simulink model "TrafegabilidadeVerticalAtivo"  (R2018a)
settings: Solver=ode3  StartTime=0.0  StopTime=60  FixedStep=0.0001  RelTol=1e-3
values from neighbouring files (symbols this model uses):
  a1 = 1    [Algoritmo_gen.m]    (also in Parametros_dissertacao_Jeff.m = 1.99; custo_gen.m)
  a2 = 100    [Algoritmo_gen.m]    (also in Parametros_dissertacao_Jeff.m = 1.988; custo_gen.m)
  b1 = 0.675    [Parametros_dissertacao_Jeff.m]
  b2 = 0.675    [Parametros_dissertacao_Jeff.m]
  bp11 = 2660    [Parametros_Susp_Ativa_GALQR.m]    (also in Parametros_dissertacao_Jeff.m)
  bp2 = 2660    [Parametros_dissertacao_Jeff.m]
  bp3 = 2660    [Parametros_dissertacao_Jeff.m]
  bs11 = 24500    [Parametros_Susp_Ativa_GALQR.m]    (also in Parametros_dissertacao_Jeff.m)
  bs2 = 10000    [Parametros_dissertacao_Jeff.m]
  bs3 = 8000    [Parametros_dissertacao_Jeff.m]
  d = 50    [Parametros_dissertacao_Jeff.m]
  fr = 0.01    [Parametros_dissertacao_Jeff.m]
  g = 9.81    [Parametros_dissertacao_Jeff.m]
  h = eig(A_cl2)    [Algoritmo_gen.m]    (also in Parametros_dissertacao_Jeff.m = 0.3; custo_gen.m)
  hcg = 1.359    [Parametros_dissertacao_Jeff.m]
  Ibyy = 66.080    (= 66.08)    [Parametros_dissertacao_Jeff.m]
  Iyy = 284800    [Parametros_dissertacao_Jeff.m]
  kp11 = 870000    [Parametros_Susp_Ativa_GALQR.m]    (also in Parametros_dissertacao_Jeff.m)
  kp2 = 770700    [Parametros_dissertacao_Jeff.m]
  kp3 = 770700    [Parametros_dissertacao_Jeff.m]
  ks11 = 55000    [Parametros_Susp_Ativa_GALQR.m]    (also in Parametros_dissertacao_Jeff.m)
  ks2 = 3220000    [Parametros_dissertacao_Jeff.m]
  ks3 = 2740000    [Parametros_dissertacao_Jeff.m]
  L = 7    [Parametros_dissertacao_Jeff.m]
  m11 = 490    [Parametros_Susp_Ativa_GALQR.m]    (also in Parametros_dissertacao_Jeff.m)
  m2 = 4500    [Algoritmo_gen.m]    (also in Parametros_dissertacao_Jeff.m = 1700; custo_gen.m; n1sistema.m = s(2))
  m3 = 1700    [Parametros_dissertacao_Jeff.m]
  ms = 18470    [Parametros_dissertacao_Jeff.m]
  ms_b = 200    [Parametros_dissertacao_Jeff.m]
  mv = 22560    [Parametros_dissertacao_Jeff.m]
  r_est = 0.542    [Parametros_dissertacao_Jeff.m]
  r_ind = (20*25.4/2+0.5*0.85*395)/1000    (= 0.421875)    [Parametros_dissertacao_Jeff.m]
(part 1 of 2)
settings Model: Creator=MA  LastModifiedBy=jeffersongomes
settings CodeAppCC: StateflowObjectComments=on
settings SimscapeCC: SimscapeNormalizeSystem=off

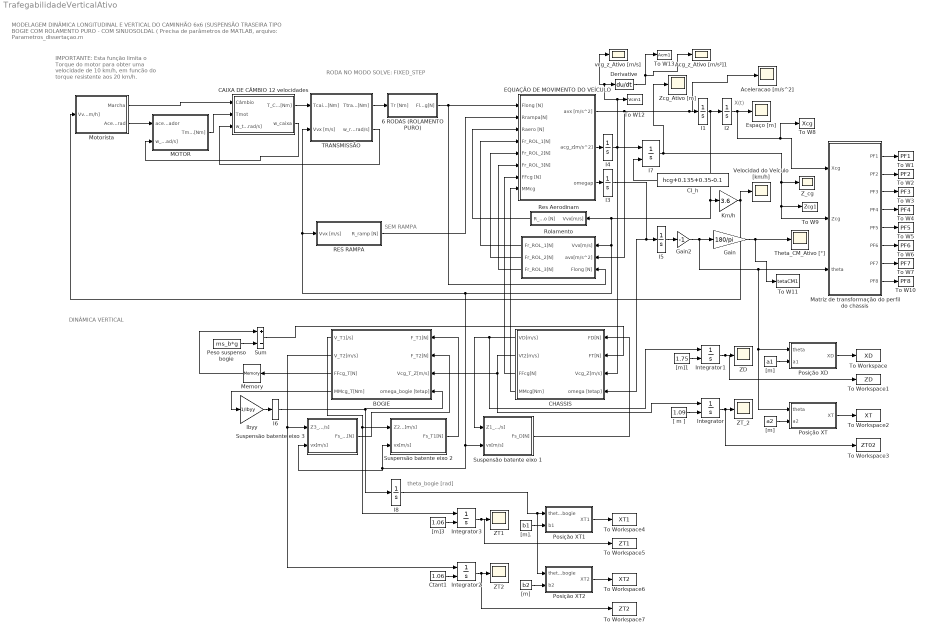
== system TrafegabilidadeVerticalAtivo ==
  note: theta_bogie [rad]
  note: SEM RAMPA
  note: RODA NO MODO SOLVE: FIXED_STEP
  note: DINÂMICA VERTICAL
  note: MODELAGEM DINÂMICA LONGITUDINAL E VERTICAL DO CAMINHÃO 6x6 (SUSPENSÃO TRASEIRA TIPO BOGIE COM ROLAMENTO PURO - COM SINUOSOLDAL
      | ( Precisa de parâmetros de MATLAB, arquivo: Parametros_dissertaçao.m
  note: X(t)
  note: IMPORTANTE:
      | Esta função limita o Torque do motor para obter uma velocidade
      | de 10 km/h, em funcão do torque resistente
      | aos 20 km/h.
  6 RODAS (ROLAMENTO PURO) : Subsystem
  Aceleracao [m/s^2] : Scope
  Acg_z_Ativo [m/s²]1 : Scope
  BOGIE : Subsystem
  CAIXA DE CÂMBIO 12 velocidades : Subsystem
  CHASSIS : Subsystem
  CI_h : Constant  Value=hcg+0.135+0.35-0.1
  Ctant1 : Constant  Value=1.06
  Derivative : Derivative
  EQUAÇÃO DE MOVIMENTO DO VEÍCULO : Subsystem
  Espaço [m] : Scope
  Gain : Gain  Gain=180/pi
  Gain2 : Gain  Gain=-1
  I1 : Integrator
  I{2..4,6} (4 alike) : Integrator  InitialCondition=eps
  I5 : Integrator  InitialCondition=-8*pi/180
  I7 : Integrator  InitialConditionSource=external  InitialCondition=1.25
  I8 : Integrator
  Ibyy : Gain  Gain=1/Ibyy
  Integrator{,1..3} (4 alike) : Integrator  InitialConditionSource=external
  Km/h : Gain  Gain=3.6
  MOTOR : Subsystem
  Matriz de transformação do perfil do chassis : MATLAB Function  TreatAsAtomicUnit=on
  Memory : Memory
  Motorista : Subsystem
  Peso suspenso bogie : Constant  Value=ms_b*g
  Posição XD : MATLAB Function  TreatAsAtomicUnit=on
  Posição XT : MATLAB Function  TreatAsAtomicUnit=on
  Posição XT1 : MATLAB Function  TreatAsAtomicUnit=on
  Posição XT2 : MATLAB Function  TreatAsAtomicUnit=on
  RES RAMPA : Subsystem
  Res Aerodinam : Subsystem
  Rolamento : Subsystem
  Sum : Sum  Inputs=+|-
  Suspensão batente eixo 1 : Subsystem
  Suspensão batente eixo 2 : Subsystem
  Suspensão batente eixo 3 : Subsystem
  TRANSMISSÃO : Subsystem
  Theta_CM_Ativo [°] : Scope
  To W1 : ToWorkspace  VariableName=PF1  SampleTime=-1
      settings: Save2DSignal=2-D array (concatenate along first dimension)
  To W10 : ToWorkspace  VariableName=PF8  SampleTime=-1
      settings: Save2DSignal=2-D array (concatenate along first dimension)
  To W11 : ToWorkspace  VariableName=tetaCM1  SampleTime=-1
      settings: Save2DSignal=2-D array (concatenate along first dimension)
  To W12 : ToWorkspace  VariableName=Vcm1  SampleTime=-1
      settings: Save2DSignal=2-D array (concatenate along first dimension)
  To W13 : ToWorkspace  VariableName=Acm1  SampleTime=-1
      settings: Save2DSignal=2-D array (concatenate along first dimension)
  To W2 : ToWorkspace  VariableName=PF2  SampleTime=-1
      settings: Save2DSignal=2-D array (concatenate along first dimension)
  To W3 : ToWorkspace  VariableName=PF3  SampleTime=-1
      settings: Save2DSignal=2-D array (concatenate along first dimension)
  To W4 : ToWorkspace  VariableName=PF4  SampleTime=-1
      settings: Save2DSignal=2-D array (concatenate along first dimension)
  To W5 : ToWorkspace  VariableName=PF5  SampleTime=-1
      settings: Save2DSignal=2-D array (concatenate along first dimension)
  To W6 : ToWorkspace  VariableName=PF6  SampleTime=-1
      settings: Save2DSignal=2-D array (concatenate along first dimension)
  To W7 : ToWorkspace  VariableName=PF7  SampleTime=-1
      settings: Save2DSignal=2-D array (concatenate along first dimension)
  To W8 : ToWorkspace  VariableName=Xcg  SampleTime=-1
      settings: Save2DSignal=2-D array (concatenate along first dimension)
  To W9 : ToWorkspace  VariableName=Zcg1  SampleTime=-1
      settings: Save2DSignal=2-D array (concatenate along first dimension)
  To Workspace : ToWorkspace  VariableName=XD  SampleTime=-1
      settings: Save2DSignal=2-D array (concatenate along first dimension)
  To Workspace1 : ToWorkspace  VariableName=ZD  SampleTime=-1
      settings: Save2DSignal=2-D array (concatenate along first dimension)
  To Workspace2 : ToWorkspace  VariableName=XT  SampleTime=-1
      settings: Save2DSignal=2-D array (concatenate along first dimension)
  To Workspace3 : ToWorkspace  VariableName=ZT02  SampleTime=-1
      settings: Save2DSignal=2-D array (concatenate along first dimension)
  To Workspace4 : ToWorkspace  VariableName=XT1  SampleTime=-1
      settings: Save2DSignal=2-D array (concatenate along first dimension)
  To Workspace5 : ToWorkspace  VariableName=ZT1  SampleTime=-1
      settings: Save2DSignal=2-D array (concatenate along first dimension)
  To Workspace6 : ToWorkspace  VariableName=XT2  SampleTime=-1
      settings: Save2DSignal=2-D array (concatenate along first dimension)
  To Workspace7 : ToWorkspace  VariableName=ZT2  SampleTime=-1
      settings: Save2DSignal=2-D array (concatenate along first dimension)
  Velocidad do Veículo [km/h] : Scope
  ZD : Scope
  ZT1 : Scope
  ZT2 : Scope
  ZT_2 : Scope
  Z_cg : Scope
  Zcg_Ativo [m] : Scope
  "[ m ] " : Constant  Value=1.09
  "[m]" : Constant  Value=a1
  "[m] " : Constant  Value=a2
  "[m]  " : Constant  Value=b2
  "[m]." : Constant  Value=b1
  "[m]1" : Constant  Value=1.75
  "[m]3" : Constant  Value=1.06
  vcg_z_Ativo [m/s] : Scope
  wires:
  I2/1 -> Matriz de transformação do perfil do chassis/1(Xcg), To W8/1, Espaço [m]/1
  MOTOR/1(Tmot[Nm]) -> CAIXA DE CÂMBIO 12 velocidades/2(Tmot)
  Motorista/1(Marcha) -> CAIXA DE CÂMBIO 12 velocidades/1(Câmbio)
  CAIXA DE CÂMBIO 12 velocidades/2(w_caixa) -> MOTOR/2(w_Trans [rad/s])
  CAIXA DE CÂMBIO 12 velocidades/1(T_Caixa[Nm]) -> TRANSMISSÃO/1(Tcaixa[Nm])
  TRANSMISSÃO/2(w_roda[rad/s]) -> CAIXA DE CÂMBIO 12 velocidades/3(w_trans[rad/s])
  RES RAMPA/1(R_ramp [N]) -> EQUAÇÃO DE MOVIMENTO DO VEÍCULO/2(Rrampa[N])
  Rolamento/1(Fr_ROL_1[N]) -> EQUAÇÃO DE MOVIMENTO DO VEÍCULO/4(Fr_ROL_1[N])
  TRANSMISSÃO/1(Ttrans[Nm]) -> 6 RODAS (ROLAMENTO PURO)/1(Tr [Nm])
  6 RODAS (ROLAMENTO PURO)/1(Flong[N]) -> EQUAÇÃO DE MOVIMENTO DO VEÍCULO/1(Flong [N]), Rolamento/3(Flong [N])
  EQUAÇÃO DE MOVIMENTO DO VEÍCULO/1(avx [m/s^2]) -> Aceleracao [m/s^2]/1, I1/1, Rolamento/2(avx[m/s^2])
  EQUAÇÃO DE MOVIMENTO DO VEÍCULO/3(omegap) -> I3/1
  I3/1 -> I5/1, CHASSIS/4(omega [tetap])
  EQUAÇÃO DE MOVIMENTO DO VEÍCULO/2(acg_z[m/s^2]) -> I4/1
  I4/1 -> I7/1, CHASSIS/3("Vcg_Z[m/s] "), vcg_z_Ativo [m/s]/1, Derivative/1, To W12/1
  CHASSIS/3("FFcg[N] ") -> EQUAÇÃO DE MOVIMENTO DO VEÍCULO/7(FFcg [N])
  CHASSIS/4(MMcg[Nm]) -> EQUAÇÃO DE MOVIMENTO DO VEÍCULO/8(MMcg)
  Suspensão batente eixo 1/1(Fs_D[N]) -> CHASSIS/1(FD[N])
  Gain/1 -> To W11/1, Theta_CM_Ativo [°]/1
  Suspensão batente eixo 2/1(Fs_T1[N]) -> BOGIE/1(F_T1[N])
  Suspensão batente eixo 3/1(Fs_T2[N]) -> BOGIE/2(F_T2[N])
  BOGIE/1("V_T1[/s] ") -> Integrator3/1, Suspensão batente eixo 2/1(Z2_p[m/s])
  BOGIE/2("V_T2[m/s] ") -> Integrator2/1, Suspensão batente eixo 3/1(Z3_p[m/s])
  Peso suspenso bogie/1 -> Sum/2
  BOGIE/3("FFcg_T[N] ") -> Memory/1
  Sum/1 -> CHASSIS/2(FT[N])
  BOGIE/4(MMcg_T[Nm]) -> Ibyy/1
  Ibyy/1 -> I6/1
  I1/1 -> I2/1, Res Aerodinam/1(Vvx[m/s]), RES RAMPA/1(Vvx [m/s]), TRANSMISSÃO/2(Vvx [m/s]), Suspensão batente eixo 3/2(vx[m/s]), Suspensão batente eixo 2/2(vx[m/s]), Suspensão batente eixo 1/2(vx[m/s]), Rolamento/1(Vvx[m/s]), Km/h/1
  Integrator/1 -> To Workspace3/1, ZT_2/1
  "[ m ] "/1 -> Integrator/2
  Integrator1/1 -> To Workspace1/1, ZD/1
  "[m]1"/1 -> Integrator1/2
  CHASSIS/1("VD[m/s] ") -> Integrator1/1, Suspensão batente eixo 1/1(Z1_p[m/s])
  Posição XD/1(XD) -> To Workspace/1
  "[m]"/1 -> Posição XD/2(a1)
  "[m] "/1 -> Posição XT/2(a2)
  Posição XT/1(XT) -> To Workspace2/1
  "[m]  "/1 -> Posição XT2/2(b2)
  Integrator2/1 -> To Workspace7/1, ZT2/1
  Posição XT1/1(XT1) -> To Workspace4/1
  Ctant1/1 -> Integrator2/2
  Integrator3/1 -> To Workspace5/1, ZT1/1
  "[m]."/1 -> Posição XT1/2(b1)
  Posição XT2/1(XT2) -> To Workspace6/1
  "[m]3"/1 -> Integrator3/2
  I7/1 -> Z_cg/1, To W9/1, Matriz de transformação do perfil do chassis/2(Zcg), Zcg_Ativo [m]/1
  I6/1 -> BOGIE/4(omega_bogie [tetap]), I8/1
  I8/1 -> Posição XT2/1(theta_bogie), Posição XT1/1(theta_bogie)
  CI_h/1 -> I7/2
  Rolamento/3(Fr_ROL_3[N]) -> EQUAÇÃO DE MOVIMENTO DO VEÍCULO/6(Fr_ROL_3[N])
  Res Aerodinam/1(R_aero [N]) -> EQUAÇÃO DE MOVIMENTO DO VEÍCULO/3(Raero [N])
  Rolamento/2(Fr_ROL_2[N]) -> EQUAÇÃO DE MOVIMENTO DO VEÍCULO/5(Fr_ROL_2[N])
  Km/h/1 -> Velocidad do Veículo [km/h]/1, Motorista/1(Vvx[Km/h])
  Matriz de transformação do perfil do chassis/1(PF1) -> To W1/1
  Matriz de transformação do perfil do chassis/2(PF2) -> To W2/1
  Matriz de transformação do perfil do chassis/6(PF6) -> To W6/1
  Matriz de transformação do perfil do chassis/7(PF7) -> To W7/1
  Matriz de transformação do perfil do chassis/5(PF5) -> To W5/1
  Matriz de transformação do perfil do chassis/4(PF4) -> To W4/1
  Matriz de transformação do perfil do chassis/3(PF3) -> To W3/1
  Matriz de transformação do perfil do chassis/8(PF8) -> To W10/1
  I5/1 -> Gain2/1
  Gain2/1 -> Matriz de transformação do perfil do chassis/3(theta), Posição XD/1(theta), Posição XT/1(theta), Gain/1
  Motorista/2(Acelerad) -> MOTOR/1(acelerador)
  CHASSIS/2("Vt2[m/s] ") -> BOGIE/3("Vcg_T_Z[m/s] "), Integrator/1
  Memory/1 -> Sum/1
  Derivative/1 -> Acg_z_Ativo [m/s²]1/1, To W13/1

== system TrafegabilidadeVerticalAtivo/6 RODAS (ROLAMENTO PURO) ==
  Tr [Nm] : Inport
  D2 : Product  Inputs=*/
  r_est[m] : Constant  Value=r_est
  Flong[N] : Outport  VectorParamsAs1DForOutWhenUnconnected=on
  wires:
  Tr [Nm]/1 -> D2/1
  r_est[m]/1 -> D2/2
  D2/1 -> Flong[N]/1

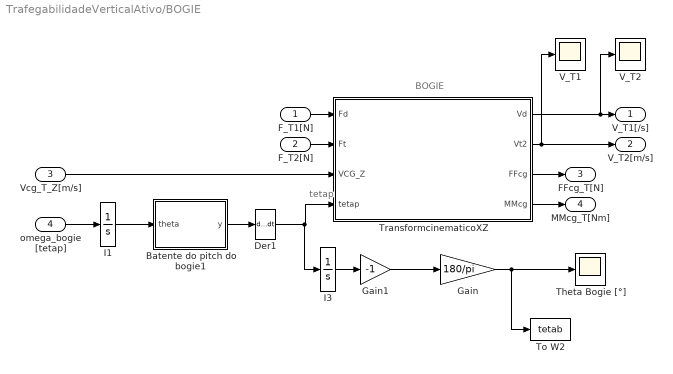
== system TrafegabilidadeVerticalAtivo/BOGIE ==
  note: BOGIE
  note: tetap
  F_T1[N] : Inport
  F_T2[N] : Inport  Port=2
  "Vcg_T_Z[m/s] " : Inport  Port=3
  omega_bogie [tetap] : Inport  Port=4
  Batente do pitch do bogie1 : MATLAB Function  TreatAsAtomicUnit=on
  Der1 : Derivative
  Gain : Gain  Gain=180/pi
  Gain1 : Gain  Gain=-1
  I1 : Integrator  InitialCondition=eps
  I3 : Integrator
  Theta Bogie [°] : Scope
  To W2 : ToWorkspace  VariableName=tetab  SampleTime=-1
      settings: Save2DSignal=2-D array (concatenate along first dimension)
  TransformcinematicoXZ : MATLAB Function  TreatAsAtomicUnit=on
  V_T1 : Scope
  V_T2 : Scope
  "V_T1[/s] " : Outport  VectorParamsAs1DForOutWhenUnconnected=on
  "V_T2[m/s] " : Outport  Port=2  VectorParamsAs1DForOutWhenUnconnected=on
  "FFcg_T[N] " : Outport  Port=3  VectorParamsAs1DForOutWhenUnconnected=on
  MMcg_T[Nm] : Outport  Port=4  VectorParamsAs1DForOutWhenUnconnected=on
  wires:
  F_T2[N]/1 -> TransformcinematicoXZ/2(Ft)
  F_T1[N]/1 -> TransformcinematicoXZ/1(Fd)
  TransformcinematicoXZ/4(MMcg) -> MMcg_T[Nm]/1
  TransformcinematicoXZ/3(FFcg) -> "FFcg_T[N] "/1
  TransformcinematicoXZ/1(Vd) -> "V_T1[/s] "/1, V_T2/1
  TransformcinematicoXZ/2(Vt2) -> "V_T2[m/s] "/1, V_T1/1
  omega_bogie [tetap]/1 -> I1/1
  I3/1 -> Gain1/1
  Gain/1 -> To W2/1, Theta Bogie [°]/1
  Der1/1 -> I3/1, TransformcinematicoXZ/4(tetap)
  Gain1/1 -> Gain/1
  "Vcg_T_Z[m/s] "/1 -> TransformcinematicoXZ/3(VCG_Z)
  I1/1 -> Batente do pitch do bogie1/1(theta)
  Batente do pitch do bogie1/1(y) -> Der1/1

== system TrafegabilidadeVerticalAtivo/CAIXA DE CÂMBIO 12 velocidades ==
  note: CAIXA DE VELOCIDADES
  Câmbio : Inport
  Tmot : Inport  Port=2
  w_trans[rad/s] : Inport  Port=3
  Product13 : Product
  Product3 : Product
  Ralações de Tran : Stateflow chart  TreatAsAtomicUnit=on
  TCaixa[Nm] : Scope
  i_caixa : Display
  i_trans : Scope
  marchas : Scope
  T_Caixa[Nm] : Outport  VectorParamsAs1DForOutWhenUnconnected=on
  w_caixa : Outport  Port=2  VectorParamsAs1DForOutWhenUnconnected=on
  wires:
  Product13/1 -> w_caixa/1
  Ralações de Tran/1(i) -> i_caixa/1, i_trans/1, Product13/1, Product3/2
  w_trans[rad/s]/1 -> Product13/2
  Tmot/1 -> Product3/1
  Câmbio/1 -> marchas/1, Ralações de Tran/1(m)
  Product3/1 -> T_Caixa[Nm]/1, TCaixa[Nm]/1

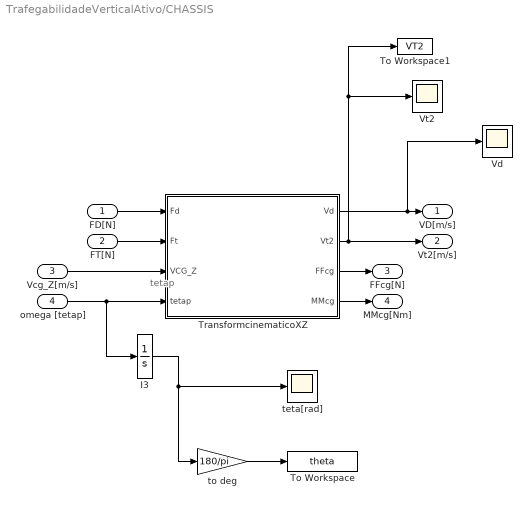
== system TrafegabilidadeVerticalAtivo/CHASSIS ==
  note: tetap
  FD[N] : Inport
  FT[N] : Inport  Port=2
  "Vcg_Z[m/s] " : Inport  Port=3
  omega [tetap] : Inport  Port=4
  I3 : Integrator
  To Workspace : ToWorkspace  VariableName=theta  SampleTime=-1
      settings: Save2DSignal=2-D array (concatenate along first dimension)
  To Workspace1 : ToWorkspace  VariableName=VT2  SampleTime=-1
      settings: Save2DSignal=2-D array (concatenate along first dimension)
  TransformcinematicoXZ : MATLAB Function  TreatAsAtomicUnit=on
  Vd : Scope
  Vt2 : Scope
  teta[rad] : Scope
  to deg : Gain  Gain=180/pi
  "VD[m/s] " : Outport  VectorParamsAs1DForOutWhenUnconnected=on
  "Vt2[m/s] " : Outport  Port=2  VectorParamsAs1DForOutWhenUnconnected=on
  "FFcg[N] " : Outport  Port=3  VectorParamsAs1DForOutWhenUnconnected=on
  MMcg[Nm] : Outport  Port=4  VectorParamsAs1DForOutWhenUnconnected=on
  wires:
  "Vcg_Z[m/s] "/1 -> TransformcinematicoXZ/3(VCG_Z)
  omega [tetap]/1 -> I3/1, TransformcinematicoXZ/4(tetap)
  TransformcinematicoXZ/2(Vt2) -> To Workspace1/1, Vt2/1, "Vt2[m/s] "/1
  TransformcinematicoXZ/1(Vd) -> Vd/1, "VD[m/s] "/1
  TransformcinematicoXZ/3(FFcg) -> "FFcg[N] "/1
  TransformcinematicoXZ/4(MMcg) -> MMcg[Nm]/1
  I3/1 -> to deg/1, teta[rad]/1
  FD[N]/1 -> TransformcinematicoXZ/1(Fd)
  FT[N]/1 -> TransformcinematicoXZ/2(Ft)
  to deg/1 -> To Workspace/1

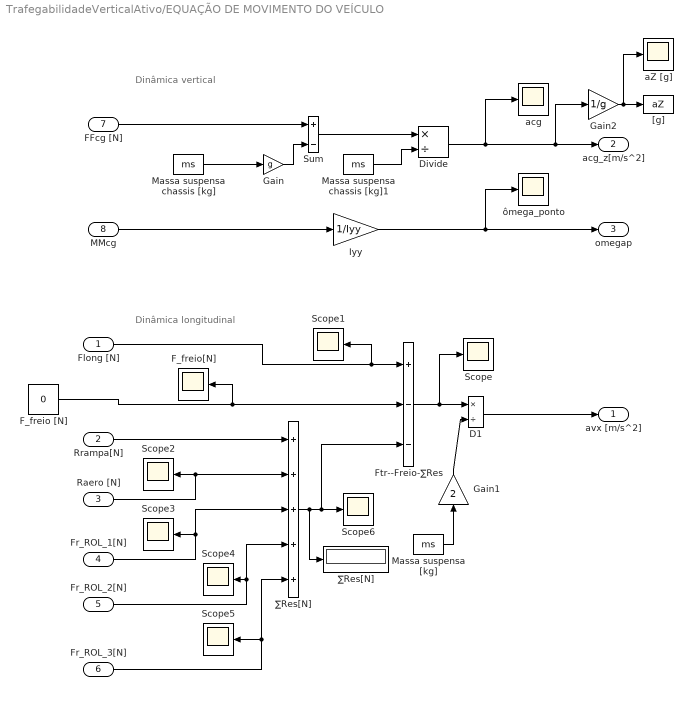
== system TrafegabilidadeVerticalAtivo/EQUAÇÃO DE MOVIMENTO DO VEÍCULO ==
  note: Dinâmica longitudinal
  note: Dinâmica vertical
  Flong [N] : Inport
  Rrampa[N] : Inport  Port=2
  Raero [N] : Inport  Port=3
  Fr_ROL_1[N] : Inport  Port=4
  Fr_ROL_2[N] : Inport  Port=5
  Fr_ROL_3[N] : Inport  Port=6
  FFcg [N] : Inport  Port=7
  MMcg : Inport  Port=8
  D1 : Product  Inputs=*/
  Divide : Product  Inputs=*/
  F_freio [N] : Constant  Value=0
  F_freio[N] : Scope
  Ftr--Freio-∑Res : Sum  Inputs=+--
  Gain : Gain  Gain=g
  Gain1 : Gain  Gain=2
  Gain2 : Gain  Gain=1/g
  Iyy : Gain  Gain=1/Iyy
  Massa suspensa [kg] : Constant  Value=ms
  Massa suspensa chassis [kg] : Constant  Value=ms
  Massa suspensa chassis [kg]1 : Constant  Value=ms
  Scope{,1..6} (7 alike) : Scope
  Sum : Sum  Inputs=+|-
  "[g]" : ToWorkspace  VariableName=aZ  SampleTime=-1
      settings: Save2DSignal=2-D array (concatenate along first dimension)
  aZ [g] : Scope
  acg : Scope
  ômega_ponto : Scope
  ∑Res[N] : Sum  Inputs=+++++
  "∑Res[N] " : Display
  avx [m/s^2] : Outport  VectorParamsAs1DForOutWhenUnconnected=on
  acg_z[m/s^2] : Outport  Port=2  VectorParamsAs1DForOutWhenUnconnected=on
  omegap : Outport  Port=3  VectorParamsAs1DForOutWhenUnconnected=on
  wires:
  Rrampa[N]/1 -> ∑Res[N]/1
  Flong [N]/1 -> Scope1/1, Ftr--Freio-∑Res/1
  Fr_ROL_2[N]/1 -> ∑Res[N]/4, Scope4/1
  ∑Res[N]/1 -> "∑Res[N] "/1, Scope6/1, Ftr--Freio-∑Res/3
  D1/1 -> avx [m/s^2]/1
  Raero [N]/1 -> ∑Res[N]/2, Scope2/1
  Fr_ROL_1[N]/1 -> ∑Res[N]/3, Scope3/1
  Ftr--Freio-∑Res/1 -> Scope/1, D1/1
  F_freio [N]/1 -> F_freio[N]/1, Ftr--Freio-∑Res/2
  Divide/1 -> acg/1, Gain2/1, acg_z[m/s^2]/1
  Iyy/1 -> omegap/1, ômega_ponto/1
  Massa suspensa [kg]/1 -> Gain1/1
  MMcg/1 -> Iyy/1
  Sum/1 -> Divide/1
  FFcg [N]/1 -> Sum/1
  Massa suspensa chassis [kg]/1 -> Gain/1
  Fr_ROL_3[N]/1 -> ∑Res[N]/5, Scope5/1
  Gain/1 -> Sum/2
  Massa suspensa chassis [kg]1/1 -> Divide/2
  Gain1/1 -> D1/2
  Gain2/1 -> aZ [g]/1, "[g]"/1

== system TrafegabilidadeVerticalAtivo/MOTOR ==
  note: MOTOR
  note: IMPORTANTE:
      | Esta função limita o Torque do motor para obter uma velocidade
      | de 10 km/h, em funcão do torque resistente
      | aos 20 km/h.
  acelerador : Inport
  w_Trans [rad/s] : Inport  Port=2
  Pmáx[kW] : Constant  Value=302
  Ralenti_Limitador : MATLAB Function  TreatAsAtomicUnit=on
  T_min [Nm] : MATLAB Function  TreatAsAtomicUnit=on
  Tmot [Nm] : Scope
  Torque motor [Nm] : MATLAB Function  TreatAsAtomicUnit=on
  to rpm : Gain  Gain=30/pi
  wPmáx[rpm] : Constant  Value=1900
  wm[rad/s] : Scope
  wm[rpm] : Scope
  Tmot[Nm] : Outport  VectorParamsAs1DForOutWhenUnconnected=on
  wires:
  Pmáx[kW]/1 -> Torque motor [Nm]/1(Pmax)
  wPmáx[rpm]/1 -> Torque motor [Nm]/2(wPmax)
  w_Trans [rad/s]/1 -> Ralenti_Limitador/1(u)
  Ralenti_Limitador/1(y) -> wm[rad/s]/1, Torque motor [Nm]/3(w), to rpm/1
  Torque motor [Nm]/1(T) -> T_min [Nm]/2(T)
  T_min [Nm]/1(Tmot) -> Tmot[Nm]/1, Tmot [Nm]/1
  acelerador/1 -> T_min [Nm]/1(acel)
  to rpm/1 -> wm[rpm]/1

== system TrafegabilidadeVerticalAtivo/Motorista ==
  note: MOTORISTA
  Vvx[Km/h] : Inport
  Acelerador : MATLAB Function  TreatAsAtomicUnit=on
  Clock : Clock
  Limitador de marcha : MATLAB Function  TreatAsAtomicUnit=on
  Scope : Scope
  Scope1 : Scope
  Seletor de marcha : Stateflow chart  TreatAsAtomicUnit=on
  To W1 : ToWorkspace  VariableName=tempo  SampleTime=-1
      settings: Save2DSignal=2-D array (concatenate along first dimension)
  To W2 : ToWorkspace  VariableName=vX  SampleTime=-1
      settings: Save2DSignal=2-D array (concatenate along first dimension)
  Marcha : Outport  VectorParamsAs1DForOutWhenUnconnected=on
  Acelerad : Outport  Port=2  VectorParamsAs1DForOutWhenUnconnected=on
  wires:
  Seletor de marcha/1(m) -> Limitador de marcha/1(m)
  Acelerador/1(y) -> Scope/1, Acelerad/1
  Clock/1 -> To W1/1, Acelerador/1(t)
  Limitador de marcha/1(marcha) -> Marcha/1, Scope1/1
  Vvx[Km/h]/1 -> To W2/1, Limitador de marcha/2(v), Acelerador/2(v), Seletor de marcha/1(v)

== system TrafegabilidadeVerticalAtivo/RES RAMPA ==
  Vvx [m/s] : Inport
  Massa do veículo [kg] : Constant  Value=mv
  P1 : Product
  R_ramp[N] : Constant  Value=0
  Rampa  [°] : Constant  Value=0
  Switch : Switch  Criteria=u2 > Threshold
  Trig : Trigonometry
  g[m/s^2] : Gain  Gain=9.81
  ° a rad : Gain  Gain=pi/180
  R_ramp [N] : Outport  VectorParamsAs1DForOutWhenUnconnected=on
  wires:
  Rampa  [°]/1 -> ° a rad/1
  Trig/1 -> P1/1
  ° a rad/1 -> Trig/1
  g[m/s^2]/1 -> P1/2
  Massa do veículo [kg]/1 -> g[m/s^2]/1
  Vvx [m/s]/1 -> Switch/2
  Switch/1 -> R_ramp [N]/1
  P1/1 -> Switch/1
  R_ramp[N]/1 -> Switch/3

== system TrafegabilidadeVerticalAtivo/Res Aerodinam ==
  Vvx[m/s] : Inport
  Area Frontal [m^2] : Constant  Value=8
  "CD [ _ ] " : Constant  Value=0.673
  Densidad do Ar  [kg/m^3) : Constant  Value=1.28
  "Ftr_t " : MATLAB Function  TreatAsAtomicUnit=on
  Scope : Scope
  R_aero [N] : Outport  VectorParamsAs1DForOutWhenUnconnected=on
  wires:
  "Ftr_t "/1(R_aero) -> Scope/1, R_aero [N]/1
  Vvx[m/s]/1 -> "Ftr_t "/4(Vv)
  Densidad do Ar  [kg/m^3)/1 -> "Ftr_t "/1(ro)
  Area Frontal [m^2]/1 -> "Ftr_t "/2(Af)
  "CD [ _ ] "/1 -> "Ftr_t "/3(Cx)

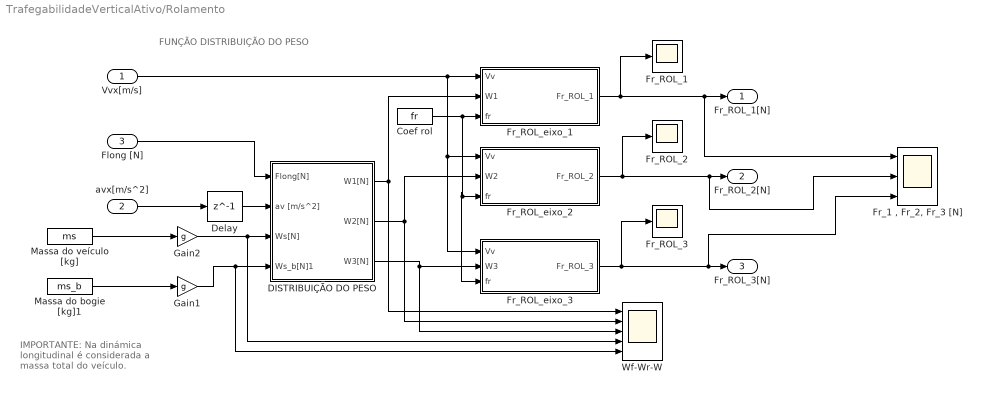
== system TrafegabilidadeVerticalAtivo/Rolamento ==
  note: IMPORTANTE:
      | Na dinámica longitudinal
      | é considerada a massa total
      | do veículo.
  note: FUNÇÃO DISTRIBUIÇÃO DO PESO
  Vvx[m/s] : Inport
  avx[m/s^2] : Inport  Port=2
  Flong [N] : Inport  Port=3
  Coef rol : Constant  Value=fr
  "DISTRIBUIÇÃO DO PESO " : Subsystem
  Delay : Delay  DelayLength=1
  "Fr_1 , Fr_2, Fr_3 [N]" : Scope  NumInputPorts=3
  Fr_ROL_1 : Scope
  Fr_ROL_2 : Scope
  Fr_ROL_3 : Scope
  Fr_ROL_eixo_1 : MATLAB Function  TreatAsAtomicUnit=on
  Fr_ROL_eixo_2 : MATLAB Function  TreatAsAtomicUnit=on
  Fr_ROL_eixo_3 : MATLAB Function  TreatAsAtomicUnit=on
  Gain1 : Gain  Gain=g
  Gain2 : Gain  Gain=g
  Massa do bogie [kg]1 : Constant  Value=ms_b
  Massa do veículo [kg] : Constant  Value=ms
  Wf-Wr-W : Scope  NumInputPorts=5
  Fr_ROL_1[N] : Outport  VectorParamsAs1DForOutWhenUnconnected=on
  Fr_ROL_2[N] : Outport  Port=2  VectorParamsAs1DForOutWhenUnconnected=on
  Fr_ROL_3[N] : Outport  Port=3  VectorParamsAs1DForOutWhenUnconnected=on
  wires:
  "DISTRIBUIÇÃO DO PESO "/2(W2[N]) -> Wf-Wr-W/2, Fr_ROL_eixo_2/2(W2)
  "DISTRIBUIÇÃO DO PESO "/1(W1[N]) -> Wf-Wr-W/1, Fr_ROL_eixo_1/2(W1)
  Vvx[m/s]/1 -> Fr_ROL_eixo_3/1(Vv), Fr_ROL_eixo_2/1(Vv), Fr_ROL_eixo_1/1(Vv)
  Fr_ROL_eixo_1/1(Fr_ROL_1) -> Fr_ROL_1/1, "Fr_1 , Fr_2, Fr_3 [N]"/1, Fr_ROL_1[N]/1
  Fr_ROL_eixo_2/1(Fr_ROL_2) -> Fr_ROL_2/1, "Fr_1 , Fr_2, Fr_3 [N]"/2, Fr_ROL_2[N]/1
  Gain2/1 -> Wf-Wr-W/4, "DISTRIBUIÇÃO DO PESO "/3(Ws[N])
  Coef rol/1 -> Fr_ROL_eixo_3/3(fr), Fr_ROL_eixo_2/3(fr), Fr_ROL_eixo_1/3(fr)
  Gain1/1 -> Wf-Wr-W/5, "DISTRIBUIÇÃO DO PESO "/4(Ws_b[N]1)
  Fr_ROL_eixo_3/1(Fr_ROL_3) -> "Fr_1 , Fr_2, Fr_3 [N]"/3, Fr_ROL_3[N]/1, Fr_ROL_3/1
  "DISTRIBUIÇÃO DO PESO "/3(W3[N]) -> Wf-Wr-W/3, Fr_ROL_eixo_3/2(W3)
  Flong [N]/1 -> "DISTRIBUIÇÃO DO PESO "/1(Flong[N])
  Massa do veículo [kg]/1 -> Gain2/1
  Massa do bogie [kg]1/1 -> Gain1/1
  avx[m/s^2]/1 -> Delay/1
  Delay/1 -> "DISTRIBUIÇÃO DO PESO "/2(av [m/s^2])

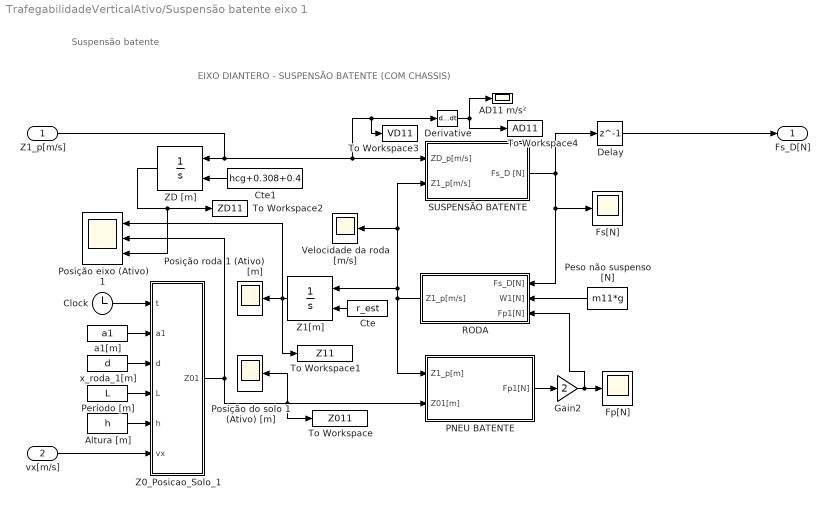
== system TrafegabilidadeVerticalAtivo/Suspensão batente eixo 1 ==
  note: Suspensão batente
  note: EIXO DIANTERO - SUSPENSÃO BATENTE (COM CHASSIS)
  Z1_p[m/s] : Inport
  vx[m/s] : Inport  Port=2
  AD11 m/s² : Scope
  Altura [m] : Constant  Value=h
  Clock : Clock
  Cte : Constant  Value=r_est  VectorParams1D=off  SampleTime=-1
  Cte1 : Constant  Value=hcg+0.308+0.4  VectorParams1D=off  SampleTime=-1
  Delay : Delay  DelayLength=1
  Derivative : Derivative
  Fp[N] : Scope
  Fs[N] : Scope
  Gain2 : Gain  Gain=2
  PNEU BATENTE : Subsystem
  Período [m] : Constant  Value=L
  Peso não suspenso [N] : Constant  Value=m11*g
  Posição do solo 1 (Ativo) [m] : Scope
  Posição roda 1 (Ativo) [m] : Scope
  Posição eixo (Ativo) 1 : Scope  NumInputPorts=3
  RODA : Subsystem
  SUSPENSÃO BATENTE : Subsystem
  To Workspace : ToWorkspace  VariableName=Z011  SampleTime=-1
      settings: Save2DSignal=2-D array (concatenate along first dimension)
  To Workspace1 : ToWorkspace  VariableName=Z11  SampleTime=-1
      settings: Save2DSignal=2-D array (concatenate along first dimension)
  To Workspace2 : ToWorkspace  VariableName=ZD11  SampleTime=-1
      settings: Save2DSignal=2-D array (concatenate along first dimension)
  To Workspace3 : ToWorkspace  VariableName=VD11  SampleTime=-1
      settings: Save2DSignal=2-D array (concatenate along first dimension)
  To Workspace4 : ToWorkspace  VariableName=AD11  SampleTime=-1
      settings: Save2DSignal=2-D array (concatenate along first dimension)
  Velocidade da roda [m/s] : Scope
  Z0_Posicao_Solo_1 : MATLAB Function  TreatAsAtomicUnit=on
  Z1[m] : Integrator  InitialConditionSource=external
  ZD [m] : Integrator  InitialConditionSource=external
  a1[m] : Constant  Value=a1
  x_roda_1[m] : Constant  Value=d
  Fs_D[N] : Outport  VectorParamsAs1DForOutWhenUnconnected=on
  wires:
  Peso não suspenso [N]/1 -> RODA/2(W1[N])
  Cte/1 -> Z1[m]/2
  SUSPENSÃO BATENTE/1(Fs_D [N]) -> RODA/1(Fs_D[N]), Fs[N]/1, Delay/1
  RODA/1(Z1_p[m/s]) -> SUSPENSÃO BATENTE/2(Z1_p[m/s]), Velocidade da roda [m/s]/1, Z1[m]/1, PNEU BATENTE/1(Z1_p[m])
  Z1[m]/1 -> Posição roda 1 (Ativo) [m]/1, Posição eixo (Ativo) 1/1, To Workspace1/1
  PNEU BATENTE/1(Fp1[N]) -> Gain2/1
  Cte1/1 -> ZD [m]/2
  vx[m/s]/1 -> Z0_Posicao_Solo_1/6(vx)
  Período [m]/1 -> Z0_Posicao_Solo_1/4(L)
  x_roda_1[m]/1 -> Z0_Posicao_Solo_1/3(d)
  Altura [m]/1 -> Z0_Posicao_Solo_1/5(h)
  Z0_Posicao_Solo_1/1(Z01) -> To Workspace/1, PNEU BATENTE/2(Z01[m]), Posição do solo 1 (Ativo) [m]/1, Posição eixo (Ativo) 1/2
  a1[m]/1 -> Z0_Posicao_Solo_1/2(a1)
  Clock/1 -> Z0_Posicao_Solo_1/1(t)
  Delay/1 -> Fs_D[N]/1
  Gain2/1 -> RODA/3(Fp1[N]), Fp[N]/1
  ZD [m]/1 -> Posição eixo (Ativo) 1/3, To Workspace2/1
  Z1_p[m/s]/1 -> ZD [m]/1, Derivative/1, To Workspace3/1, SUSPENSÃO BATENTE/1(ZD_p[m/s])
  Derivative/1 -> To Workspace4/1, AD11 m/s²/1

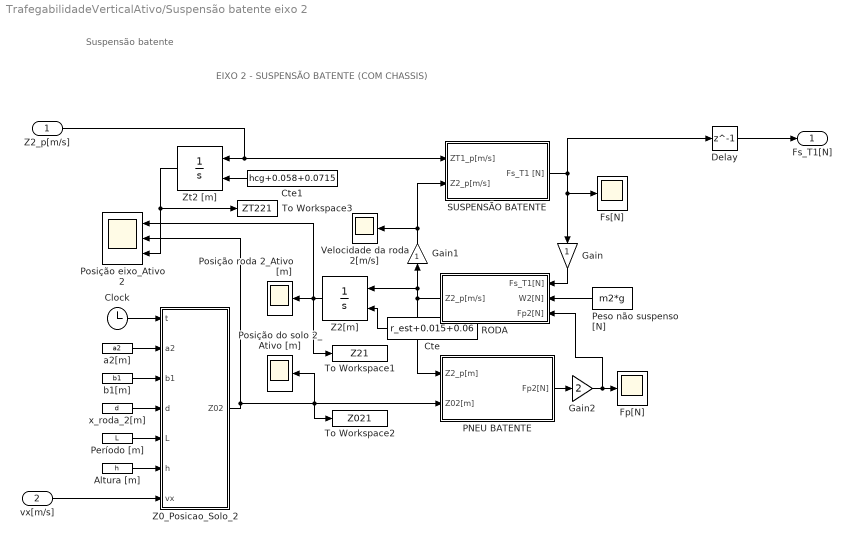
== system TrafegabilidadeVerticalAtivo/Suspensão batente eixo 2 ==
  note: EIXO 2 - SUSPENSÃO BATENTE (COM CHASSIS)
  note: Suspensão batente
  Z2_p[m/s] : Inport
  vx[m/s] : Inport  Port=2
  Altura [m] : Constant  Value=h
  Clock : Clock
  Cte : Constant  Value=r_est+0.015+0.06  VectorParams1D=off  SampleTime=-1
  Cte1 : Constant  Value=hcg+0.058+0.0715  VectorParams1D=off  SampleTime=-1
  Delay : Delay  DelayLength=1
  Fp[N] : Scope
  Fs[N] : Scope
  Gain : Gain
  Gain1 : Gain
  Gain2 : Gain  Gain=2
  PNEU BATENTE : Subsystem
  Período [m] : Constant  Value=L
  Peso não suspenso [N] : Constant  Value=m2*g
  Posição do solo 2_Ativo [m] : Scope
  Posição roda 2_Ativo [m] : Scope
  Posição eixo_Ativo 2 : Scope  NumInputPorts=3
  RODA : Subsystem
  SUSPENSÃO BATENTE : Subsystem
  To Workspace1 : ToWorkspace  VariableName=Z21  SampleTime=-1
      settings: Save2DSignal=2-D array (concatenate along first dimension)
  To Workspace2 : ToWorkspace  VariableName=Z021  SampleTime=-1
      settings: Save2DSignal=2-D array (concatenate along first dimension)
  To Workspace3 : ToWorkspace  VariableName=ZT221  SampleTime=-1
      settings: Save2DSignal=2-D array (concatenate along first dimension)
  Velocidade da roda 2[m/s] : Scope
  Z0_Posicao_Solo_2 : MATLAB Function  TreatAsAtomicUnit=on
  Z2[m] : Integrator  InitialConditionSource=external
  Zt2 [m] : Integrator  InitialConditionSource=external
  a2[m] : Constant  Value=a2
  b1[m] : Constant  Value=b1
  x_roda_2[m] : Constant  Value=d
  Fs_T1[N] : Outport  VectorParamsAs1DForOutWhenUnconnected=on
  wires:
  Cte1/1 -> Zt2 [m]/2
  Zt2 [m]/1 -> To Workspace3/1, Posição eixo_Ativo 2/3
  PNEU BATENTE/1(Fp2[N]) -> Gain2/1
  Z2[m]/1 -> Posição eixo_Ativo 2/1, Posição roda 2_Ativo [m]/1, To Workspace1/1
  Gain1/1 -> Velocidade da roda 2[m/s]/1, SUSPENSÃO BATENTE/2(Z2_p[m/s])
  RODA/1(Z2_p[m/s]) -> PNEU BATENTE/1(Z2_p[m]), Z2[m]/1, Gain1/1
  Gain/1 -> RODA/1(Fs_T1[N])
  Cte/1 -> Z2[m]/2
  Z2_p[m/s]/1 -> SUSPENSÃO BATENTE/1(ZT1_p[m/s]), Zt2 [m]/1
  Peso não suspenso [N]/1 -> RODA/2(W2[N])
  SUSPENSÃO BATENTE/1(Fs_T1 [N]) -> Delay/1, Gain/1, Fs[N]/1
  Período [m]/1 -> Z0_Posicao_Solo_2/5(L)
  Z0_Posicao_Solo_2/1(Z02) -> Posição eixo_Ativo 2/2, To Workspace2/1, Posição do solo 2_Ativo [m]/1, PNEU BATENTE/2(Z02[m])
  Altura [m]/1 -> Z0_Posicao_Solo_2/6(h)
  vx[m/s]/1 -> Z0_Posicao_Solo_2/7(vx)
  x_roda_2[m]/1 -> Z0_Posicao_Solo_2/4(d)
  b1[m]/1 -> Z0_Posicao_Solo_2/3(b1)
  a2[m]/1 -> Z0_Posicao_Solo_2/2(a2)
  Clock/1 -> Z0_Posicao_Solo_2/1(t)
  Delay/1 -> Fs_T1[N]/1
  Gain2/1 -> Fp[N]/1, RODA/3(Fp2[N])

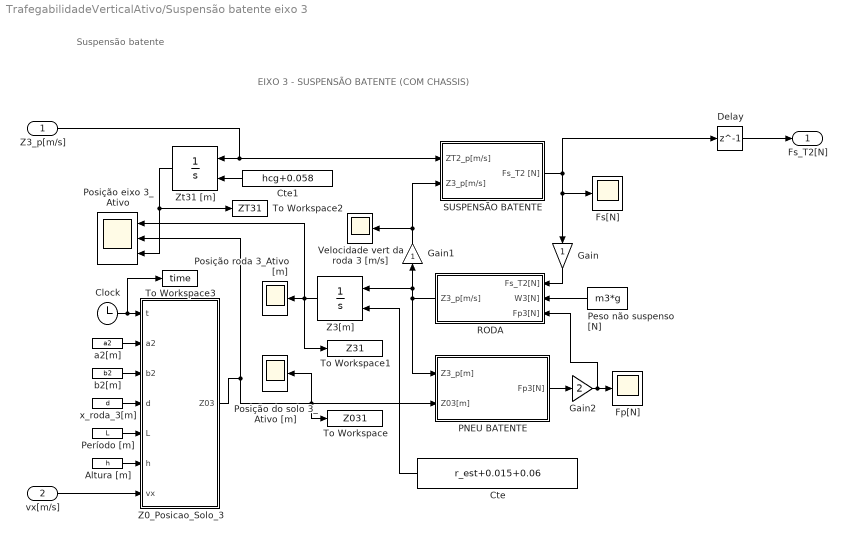
== system TrafegabilidadeVerticalAtivo/Suspensão batente eixo 3 ==
  note: Suspensão batente
  note: EIXO 3 - SUSPENSÃO BATENTE (COM CHASSIS)
  Z3_p[m/s] : Inport
  vx[m/s] : Inport  Port=2
  Altura [m] : Constant  Value=h
  Clock : Clock
  Cte : Constant  Value=r_est+0.015+0.06  VectorParams1D=off  SampleTime=-1
  Cte1 : Constant  Value=hcg+0.058  VectorParams1D=off  SampleTime=-1
  Delay : Delay  DelayLength=1
  Fp[N] : Scope
  Fs[N] : Scope
  Gain : Gain
  Gain1 : Gain
  Gain2 : Gain  Gain=2
  PNEU BATENTE : Subsystem
  Período [m] : Constant  Value=L
  Peso não suspenso [N] : Constant  Value=m3*g
  Posição do solo 3_Ativo [m] : Scope
  Posição roda 3_Ativo [m] : Scope
  Posição eixo 3_Ativo : Scope  NumInputPorts=3
  RODA : Subsystem
  SUSPENSÃO BATENTE : Subsystem
  To Workspace : ToWorkspace  VariableName=Z031  SampleTime=-1
      settings: Save2DSignal=2-D array (concatenate along first dimension)
  To Workspace1 : ToWorkspace  VariableName=Z31  SampleTime=-1
      settings: Save2DSignal=2-D array (concatenate along first dimension)
  To Workspace2 : ToWorkspace  VariableName=ZT31  SampleTime=-1
      settings: Save2DSignal=2-D array (concatenate along first dimension)
  To Workspace3 : ToWorkspace  VariableName=time  SampleTime=-1
      settings: Save2DSignal=2-D array (concatenate along first dimension)
  Velocidade vert da roda 3 [m/s] : Scope
  Z0_Posicao_Solo_3 : MATLAB Function  TreatAsAtomicUnit=on
  Z3[m] : Integrator  InitialConditionSource=external
  Zt31 [m] : Integrator  InitialConditionSource=external
  a2[m] : Constant  Value=a2
  b2[m] : Constant  Value=b2
  x_roda_3[m] : Constant  Value=d
  Fs_T2[N] : Outport  VectorParamsAs1DForOutWhenUnconnected=on
  wires:
  SUSPENSÃO BATENTE/1(Fs_T2 [N]) -> Fs[N]/1, Gain/1, Delay/1
  Peso não suspenso [N]/1 -> RODA/2(W3[N])
  Z3_p[m/s]/1 -> Zt31 [m]/1, SUSPENSÃO BATENTE/1(ZT2_p[m/s])
  Cte/1 -> Z3[m]/2
  Gain/1 -> RODA/1(Fs_T2[N])
  RODA/1(Z3_p[m/s]) -> Gain1/1, Z3[m]/1, PNEU BATENTE/1(Z3_p[m])
  Gain1/1 -> SUSPENSÃO BATENTE/2(Z3_p[m/s]), Velocidade vert da roda 3 [m/s]/1
  Z3[m]/1 -> Posição roda 3_Ativo [m]/1, Posição eixo 3_Ativo/1, To Workspace1/1
  PNEU BATENTE/1(Fp3[N]) -> Gain2/1
  Zt31 [m]/1 -> To Workspace2/1, Posição eixo 3_Ativo/3
  Cte1/1 -> Zt31 [m]/2
  Período [m]/1 -> Z0_Posicao_Solo_3/5(L)
  Z0_Posicao_Solo_3/1(Z03) -> Posição eixo 3_Ativo/2, To Workspace/1, PNEU BATENTE/2(Z03[m]), Posição do solo 3_Ativo [m]/1
  vx[m/s]/1 -> Z0_Posicao_Solo_3/7(vx)
  x_roda_3[m]/1 -> Z0_Posicao_Solo_3/4(d)
  Clock/1 -> To Workspace3/1, Z0_Posicao_Solo_3/1(t)
  Altura [m]/1 -> Z0_Posicao_Solo_3/6(h)
  a2[m]/1 -> Z0_Posicao_Solo_3/2(a2)
  b2[m]/1 -> Z0_Posicao_Solo_3/3(b2)
  Delay/1 -> Fs_T2[N]/1
  Gain2/1 -> RODA/3(Fp3[N]), Fp[N]/1

== system TrafegabilidadeVerticalAtivo/TRANSMISSÃO ==
  note: TRANSMISSÃO
  Tcaixa[Nm] : Inport
  Vvx [m/s] : Inport  Port=2
  "Desmultiplicacao " : Gain  Gain=3.96
  Divide2 : Product  Inputs=*/
  Multiplicacão i_n : Gain  Gain=3.96
  Scope : Scope
  r_roda[m] : Constant  Value=r_est
  Ttrans[Nm] : Outport  VectorParamsAs1DForOutWhenUnconnected=on
  w_roda[rad/s] : Outport  Port=2  VectorParamsAs1DForOutWhenUnconnected=on
  wires:
  Multiplicacão i_n/1 -> Scope/1, Ttrans[Nm]/1  "T_roda"
  Tcaixa[Nm]/1 -> Multiplicacão i_n/1
  "Desmultiplicacao "/1 -> w_roda[rad/s]/1
  Divide2/1 -> "Desmultiplicacao "/1  "w_roda"
  Vvx [m/s]/1 -> Divide2/1
  r_roda[m]/1 -> Divide2/2

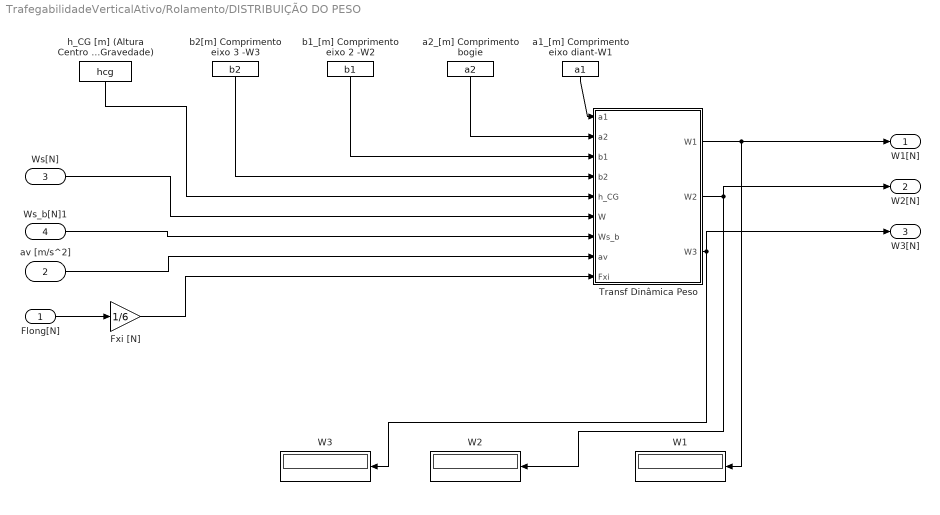
== system TrafegabilidadeVerticalAtivo/Rolamento/DISTRIBUIÇÃO DO PESO  ==
  Flong[N] : Inport
  av [m/s^2] : Inport  Port=2
  Ws[N] : Inport  Port=3
  Ws_b[N]1 : Inport  Port=4
  Fxi [N] : Gain  Gain=1/6
  Transf Dinâmica Peso : MATLAB Function  TreatAsAtomicUnit=on
  W1 : Display
  W2 : Display
  W3 : Display
  a1_[m] Comprimento eixo diant-W1 : Constant  Value=a1
  "a2_[m] Comprimento bogie " : Constant  Value=a2
  b1_[m] Comprimento eixo 2 -W2 : Constant  Value=b1
  b2[m] Comprimento eixo 3 -W3 : Constant  Value=b2
  h_CG [m] (Altura Centro de Gravedade) : Constant  Value=hcg
  W1[N] : Outport  VectorParamsAs1DForOutWhenUnconnected=on
  W2[N] : Outport  Port=2  VectorParamsAs1DForOutWhenUnconnected=on
  W3[N] : Outport  Port=3  VectorParamsAs1DForOutWhenUnconnected=on
  wires:
  Transf Dinâmica Peso/2(W2) -> W2/1, W2[N]/1
  Transf Dinâmica Peso/1(W1) -> W1/1, W1[N]/1
  Ws[N]/1 -> Transf Dinâmica Peso/6(W)
  av [m/s^2]/1 -> Transf Dinâmica Peso/8(av)
  "a2_[m] Comprimento bogie "/1 -> Transf Dinâmica Peso/2(a2)
  h_CG [m] (Altura Centro de Gravedade)/1 -> Transf Dinâmica Peso/5(h_CG)
  a1_[m] Comprimento eixo diant-W1/1 -> Transf Dinâmica Peso/1(a1)
  b1_[m] Comprimento eixo 2 -W2/1 -> Transf Dinâmica Peso/3(b1)
  b2[m] Comprimento eixo 3 -W3/1 -> Transf Dinâmica Peso/4(b2)
  Ws_b[N]1/1 -> Transf Dinâmica Peso/7(Ws_b)
  Transf Dinâmica Peso/3(W3) -> W3/1, W3[N]/1
  Flong[N]/1 -> Fxi [N]/1
  Fxi [N]/1 -> Transf Dinâmica Peso/9(Fxi)

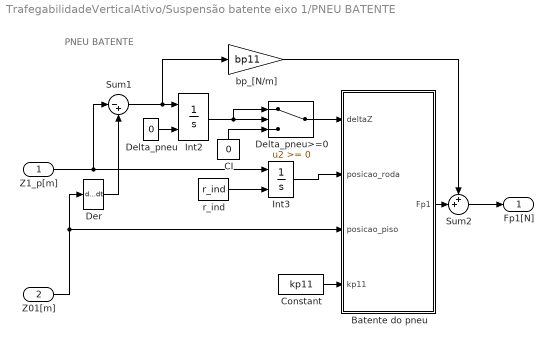
== system TrafegabilidadeVerticalAtivo/Suspensão batente eixo 1/PNEU BATENTE ==
  note: PNEU BATENTE
  Z1_p[m] : Inport
  Z01[m] : Inport  Port=2
  Batente do pneu : MATLAB Function  TreatAsAtomicUnit=on
  CI : Constant  Value=0
  Constant : Constant  Value=kp11
  Delta_pneu : Constant  Value=0
  Delta_pneu>=0 : Switch
  Der : Derivative
  Int2 : Integrator  InitialConditionSource=external
  Int3 : Integrator  InitialConditionSource=external
  Sum1 : Sum  Inputs=|-+
  Sum2 : Sum  Inputs=++|
  bp_[N/m] : Gain  Gain=bp11
  r_ind : Constant  Value=r_ind
  Fp1[N] : Outport  VectorParamsAs1DForOutWhenUnconnected=on
  wires:
  Z1_p[m]/1 -> Sum1/1, Int3/1
  Delta_pneu/1 -> Int2/2
  Sum1/1 -> bp_[N/m]/1, Int2/1
  Sum2/1 -> Fp1[N]/1
  Der/1 -> Sum1/2
  bp_[N/m]/1 -> Sum2/1
  Batente do pneu/1(Fp1) -> Sum2/2
  Int3/1 -> Batente do pneu/2(posicao_roda)
  Z01[m]/1 -> Der/1, Batente do pneu/3(posicao_piso)
  r_ind/1 -> Int3/2
  Int2/1 -> Delta_pneu>=0/1, Delta_pneu>=0/2
  CI/1 -> Delta_pneu>=0/3
  Delta_pneu>=0/1 -> Batente do pneu/1(deltaZ)
  Constant/1 -> Batente do pneu/4(kp11)

== system TrafegabilidadeVerticalAtivo/Suspensão batente eixo 1/RODA ==
  note: RODA 1
  Fs_D[N] : Inport
  W1[N] : Inport  Port=2
  Fp1[N] : Inport  Port=3
  Constant : Constant  Value=m11
  Divide : Product  Inputs=*/
  Int : Integrator  InitialCondition=eps
  Sum4 : Sum  Inputs=|+--
  Z1_p[m/s] : Outport  VectorParamsAs1DForOutWhenUnconnected=on
  wires:
  W1[N]/1 -> Sum4/3
  Fs_D[N]/1 -> Sum4/2
  Fp1[N]/1 -> Sum4/1
  Divide/1 -> Int/1
  Int/1 -> Z1_p[m/s]/1
  Sum4/1 -> Divide/1
  Constant/1 -> Divide/2

== system TrafegabilidadeVerticalAtivo/Suspensão batente eixo 1/SUSPENSÃO BATENTE ==
  note: bs=(800Ns/m ~ 3000Ns/m)
  note: SUSPENSÃO 1 - BATENTE
  ZD_p[m/s] : Inport
  Z1_p[m/s] : Inport  Port=2
  Amortecedor : Gain  Gain=bs11
  Batente da suspensão : MATLAB Function  TreatAsAtomicUnit=on
  Cte : Constant  Value=ks11
  In1 : Integrator  InitialCondition=eps
  Sum : Sum  Inputs=|++
  Sum2 : Sum  Inputs=|-+
  Fs_D [N] : Outport  VectorParamsAs1DForOutWhenUnconnected=on
  wires:
  Sum2/1 -> Amortecedor/1, In1/1
  Z1_p[m/s]/1 -> Sum2/2
  ZD_p[m/s]/1 -> Sum2/1
  In1/1 -> Batente da suspensão/2(DeltaZ)
  Amortecedor/1 -> Sum/2
  Sum/1 -> Fs_D [N]/1
  Batente da suspensão/1(FK1) -> Sum/1
  Cte/1 -> Batente da suspensão/1(ks11)

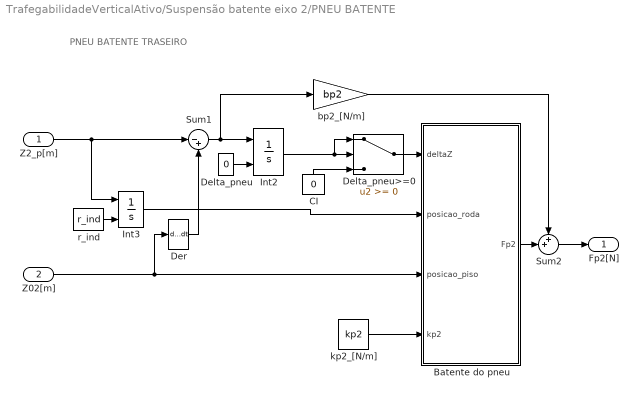
== system TrafegabilidadeVerticalAtivo/Suspensão batente eixo 2/PNEU BATENTE ==
  note: PNEU BATENTE TRASEIRO
  Z2_p[m] : Inport
  Z02[m] : Inport  Port=2
  Batente do pneu : MATLAB Function  TreatAsAtomicUnit=on
  CI : Constant  Value=0
  Delta_pneu : Constant  Value=0
  Delta_pneu>=0 : Switch
  Der : Derivative
  Int2 : Integrator  InitialConditionSource=external
  Int3 : Integrator  InitialConditionSource=external
  Sum1 : Sum  Inputs=|-+
  Sum2 : Sum  Inputs=++|
  bp2_[N/m] : Gain  Gain=bp2
  kp2_[N/m] : Constant  Value=kp2
  r_ind : Constant  Value=r_ind
  Fp2[N] : Outport  VectorParamsAs1DForOutWhenUnconnected=on
  wires:
  kp2_[N/m]/1 -> Batente do pneu/4(kp2)
  Delta_pneu>=0/1 -> Batente do pneu/1(deltaZ)
  CI/1 -> Delta_pneu>=0/3
  Int2/1 -> Delta_pneu>=0/2, Delta_pneu>=0/1
  r_ind/1 -> Int3/2
  Z02[m]/1 -> Der/1, Batente do pneu/3(posicao_piso)
  Int3/1 -> Batente do pneu/2(posicao_roda)
  Batente do pneu/1(Fp2) -> Sum2/2
  bp2_[N/m]/1 -> Sum2/1
  Der/1 -> Sum1/2
  Sum2/1 -> Fp2[N]/1
  Sum1/1 -> Int2/1, bp2_[N/m]/1
  Delta_pneu/1 -> Int2/2
  Z2_p[m]/1 -> Sum1/1, Int3/1

== system TrafegabilidadeVerticalAtivo/Suspensão batente eixo 2/RODA ==
  note: RODA 2
  Fs_T1[N] : Inport
  W2[N] : Inport  Port=2
  Fp2[N] : Inport  Port=3
  Constant : Constant  Value=m2
  Divide : Product  Inputs=*/
  In2 : Integrator
  Scope : Scope
  Sum4 : Sum  Inputs=|+--
  Z2_p[m/s] : Outport  VectorParamsAs1DForOutWhenUnconnected=on
  wires:
  Sum4/1 -> Divide/1
  In2/1 -> Z2_p[m/s]/1
  Divide/1 -> In2/1
  Fp2[N]/1 -> Sum4/1, Scope/1
  Fs_T1[N]/1 -> Sum4/2
  W2[N]/1 -> Sum4/3
  Constant/1 -> Divide/2

== system TrafegabilidadeVerticalAtivo/Suspensão batente eixo 2/SUSPENSÃO BATENTE ==
  note: SUSPENSÃO 2 - BATENTE
  note: bs=(800Ns/m ~ 3000Ns/m)
  ZT1_p[m/s] : Inport
  Z2_p[m/s] : Inport  Port=2
  Amortecedor : Gain  Gain=bs2
  Batente da suspensão : MATLAB Function  TreatAsAtomicUnit=on
  Cte : Constant  Value=ks2
  In1 : Integrator  InitialCondition=eps
  Sum : Sum  Inputs=|++
  Sum2 : Sum  Inputs=|-+
  Fs_T1 [N] : Outport  VectorParamsAs1DForOutWhenUnconnected=on
  wires:
  Cte/1 -> Batente da suspensão/1(ks2)
  Sum/1 -> Fs_T1 [N]/1
  Amortecedor/1 -> Sum/2
  ZT1_p[m/s]/1 -> Sum2/1
  Z2_p[m/s]/1 -> Sum2/2
  Sum2/1 -> Amortecedor/1, In1/1
  In1/1 -> Batente da suspensão/2(DeltaZ)
  Batente da suspensão/1(FK2) -> Sum/1

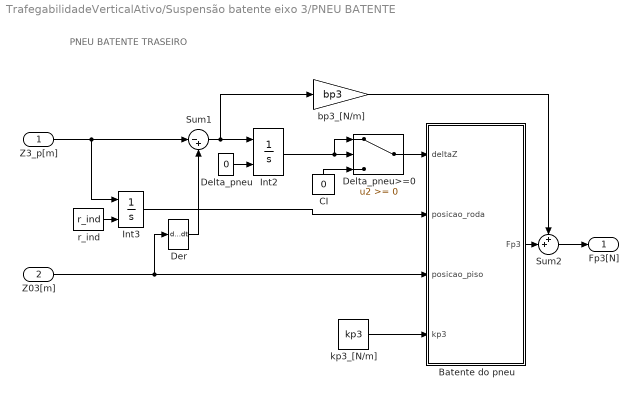
== system TrafegabilidadeVerticalAtivo/Suspensão batente eixo 3/PNEU BATENTE ==
  note: PNEU BATENTE TRASEIRO
  Z3_p[m] : Inport
  Z03[m] : Inport  Port=2
  Batente do pneu : MATLAB Function  TreatAsAtomicUnit=on
  CI : Constant  Value=0
  Delta_pneu : Constant  Value=0
  Delta_pneu>=0 : Switch
  Der : Derivative
  Int2 : Integrator  InitialConditionSource=external
  Int3 : Integrator  InitialConditionSource=external
  Sum1 : Sum  Inputs=|-+
  Sum2 : Sum  Inputs=++|
  bp3_[N/m] : Gain  Gain=bp3
  kp3_[N/m] : Constant  Value=kp3
  r_ind : Constant  Value=r_ind
  Fp3[N] : Outport  VectorParamsAs1DForOutWhenUnconnected=on
  wires:
  Z3_p[m]/1 -> Int3/1, Sum1/1
  Delta_pneu/1 -> Int2/2
  Sum1/1 -> bp3_[N/m]/1, Int2/1
  Sum2/1 -> Fp3[N]/1
  Der/1 -> Sum1/2
  bp3_[N/m]/1 -> Sum2/1
  Batente do pneu/1(Fp3) -> Sum2/2
  Int3/1 -> Batente do pneu/2(posicao_roda)
  Z03[m]/1 -> Batente do pneu/3(posicao_piso), Der/1
  r_ind/1 -> Int3/2
  Int2/1 -> Delta_pneu>=0/1, Delta_pneu>=0/2
  CI/1 -> Delta_pneu>=0/3
  Delta_pneu>=0/1 -> Batente do pneu/1(deltaZ)
  kp3_[N/m]/1 -> Batente do pneu/4(kp3)

== system TrafegabilidadeVerticalAtivo/Suspensão batente eixo 3/RODA ==
  note: RODA 3
  Fs_T2[N] : Inport
  W3[N] : Inport  Port=2
  Fp3[N] : Inport  Port=3
  Constant : Constant  Value=m3
  Divide : Product  Inputs=*/
  In2 : Integrator
  Scope : Scope
  Sum4 : Sum  Inputs=|+--
  Z3_p[m/s] : Outport  VectorParamsAs1DForOutWhenUnconnected=on
  wires:
  W3[N]/1 -> Sum4/3
  Fs_T2[N]/1 -> Sum4/2
  Fp3[N]/1 -> Scope/1, Sum4/1
  Divide/1 -> In2/1
  In2/1 -> Z3_p[m/s]/1
  Sum4/1 -> Divide/1
  Constant/1 -> Divide/2

== system TrafegabilidadeVerticalAtivo/Suspensão batente eixo 3/SUSPENSÃO BATENTE ==
  note: bs=(800Ns/m ~ 3000Ns/m)
  note: SUSPENSÃO 3 - BATENTE
  ZT2_p[m/s] : Inport
  Z3_p[m/s] : Inport  Port=2
  Amortecedor : Gain  Gain=bs3
  Batente da suspensão : MATLAB Function  TreatAsAtomicUnit=on
  Cte : Constant  Value=ks3
  In1 : Integrator  InitialCondition=eps
  Sum : Sum  Inputs=|++
  Sum2 : Sum  Inputs=|-+
  Fs_T2 [N] : Outport  VectorParamsAs1DForOutWhenUnconnected=on
  wires:
  Sum2/1 -> Amortecedor/1, In1/1
  Z3_p[m/s]/1 -> Sum2/2
  ZT2_p[m/s]/1 -> Sum2/1
  In1/1 -> Batente da suspensão/2(DeltaZ)
  Amortecedor/1 -> Sum/2
  Sum/1 -> Fs_T2 [N]/1
  Batente da suspensão/1(FK3) -> Sum/1
  Cte/1 -> Batente da suspensão/1(ks3)

== matlab function TrafegabilidadeVerticalAtivo/MOTOR/Ralenti_Limitador ==
  data: u input; y output
function y = fcn(u)  %CAMINHÃO
%u [rad/s]
w=u*30/pi;

if w<1000    %w[rpm] O MOTOR FICA EM RALENTI
    y=1000*pi/30; % [rad/s] 
else
    if w>1300   %w[rpm] w maximo MOTOR ECONOMICO
        y=1300*pi/30; % [rad/s] 
    else 
      y=u; % [rad/s] 
    end
end
end

== matlab function TrafegabilidadeVerticalAtivo/Motorista/Acelerador ==
  data: t input; y output; v input
function y=fcn(t,v)

if t>=0 
    y=1;
    if v>=10;%15  SI V=15 KM/H SE GOLPEA Y LUEGO ESTABILIZA
       y=0.3;
    end
 else
    y=0;
end
end

== stateflow chart TrafegabilidadeVerticalAtivo/CAIXA DE CÂMBIO 12 velocidades/Ralações de Tran ==
  state neutro
    entry: i=0;
  state Primeira_1
    entry: i=11.32;
  state Segunda_2
    entry: i=9.16;
  state Terceira_3
    entry: i=7.19;
  state Quarta_4
    entry: i=5.82;
  state Quinta_5
    entry: i=4.63;
  state Sexta_6
    entry: i=3.75;
  state Decima_12
    entry: i=1;
  state Decima_11
    entry: i=1.24;
  state Decima_10
    entry: i=1.55;
  state Nona_9
    entry: i=1.92;
  state Oitava_8
    entry: i=2.44;
  state Setima_7
    entry: i=3.02;
  note: ?
  note: ?
  (default) -> neutro
  neutro -> Primeira_1 : [m==1]
  Primeira_1 -> Segunda_2 [order 2] : [m==2]
  Segunda_2 -> Terceira_3 [order 2] : [m==3]
  Terceira_3 -> Quarta_4 [order 2] : [m==4]
  Quarta_4 -> Quinta_5 [order 2] : [m==5]
  Quinta_5 -> Sexta_6 [order 1] : [m==6]
  Setima_7 -> Sexta_6 [order 2] : [m<7]
  Sexta_6 -> Setima_7 [order 2] : [m==7]
  Primeira_1 -> neutro [order 1] : [m<1]
  Segunda_2 -> Primeira_1 [order 1] : [m<2]
  Terceira_3 -> Segunda_2 [order 1] : [m<3]
  Quarta_4 -> Terceira_3 [order 1] : [m<4]
  Quinta_5 -> Quarta_4 [order 2] : [m<5]
  Sexta_6 -> Quinta_5 [order 1] : [m<6]
  Decima_11 -> Decima_12 [order 2] : [m==12]
  Decima_10 -> Decima_11 [order 2] : [m==11]
  Nona_9 -> Decima_10 [order 2] : [m==10]
  Oitava_8 -> Nona_9 [order 2] : [m==9]
  Setima_7 -> Oitava_8 [order 1] : [m==8]
  Decima_12 -> Decima_11 : [m<12]
  Decima_11 -> Decima_10 [order 1] : [m<11]
  Decima_10 -> Nona_9 [order 1] : [m<10]
  Nona_9 -> Oitava_8 [order 1] : [m<9]
  Oitava_8 -> Setima_7 [order 1] : [m<8]
  data: i output; m input

== matlab function TrafegabilidadeVerticalAtivo/Suspensão batente eixo 3/PNEU BATENTE/Batente do pneu ==
  data: deltaZ input; posicao_roda input; posicao_piso input; Fp3 output; kp3 input
function Fp3= fcn(deltaZ, posicao_roda, posicao_piso,kp3)
%% Entradas: deltaZ
%%           
%% Saida: FORÇA DO PNEU [N]
%% ________________________________________________________________________

%kp3=Constante elástica (160000N/m ~ 250000N/m); PNEU(205/50/R15)

Zp=0.1975; %Altura do pneu [m]  (395/85R20)

r_ind=0.4515; %Raio indeformavel[m];  R_ind[m]=r_aro[m]+hp[m]

kp_batente=9e+06; %Faz o pneu rigido.
%%
if deltaZ>=0.95*Zp      %Deflexão maxima.
  
    kp3=kp_batente; %Faz o pneu rigido.

end

if posicao_roda-posicao_piso>r_ind %Perdida de contato
    
    Fp3=0;
    
else

    Fp3=kp3*deltaZ;%Contato normal
    
end

== matlab function TrafegabilidadeVerticalAtivo/BOGIE/Batente do pitch do bogie1 ==
  data: theta input; y output
% Sistema de Suspensão - Modelos Passivo e Semiativo
% Autor: Jefferson Gomes de Carvalho Souza
function y = fcn(theta)
theta_deg=theta*180/pi;
if theta_deg>=20 
    y=20;
else
    if theta_deg<=-20 
    y = -20*pi/180;
    else
        y=theta;
    end
end
end

== matlab function TrafegabilidadeVerticalAtivo/Rolamento/Fr_ROL_eixo_2 ==
  data: Vv input; W2 input; Fr_ROL_2 output; fr input
function Fr_ROL_2 = fcn(Vv,W2,fr)
%fr:Coeficiente de rolamento
theta=0;% Rampa em grados
%_________________________________________________________%
%____________CONDIÇÃO INICIAL DE ROLAMENTO________________%
if Vv>0   
  %__________FORÇA RESITENTE AO ROLAMENTO___________________%
 Fr_ROL_2 =fr*W2*cos(theta*pi/180);
else
    Fr_ROL_2=0;
end
end

== matlab function TrafegabilidadeVerticalAtivo/Rolamento/Fr_ROL_eixo_1 ==
  data: Vv input; W1 input; Fr_ROL_1 output; fr input
function Fr_ROL_1 = fcn(Vv,W1,fr)
%fr:Coeficiente de rolamento
theta=0;% Rampa em grados
%_________________________________________________________%
%___CONDIÇÃO INICIAL DE ROLAMENTO________________%
if Vv>0
 Fr_ROL_1 =fr*W1*cos(theta*pi/180);
else
    Fr_ROL_1=0;
end
end

== matlab function TrafegabilidadeVerticalAtivo/Res Aerodinam/Ftr_t  ==
  data: ro input; Af input; R_aero output; Cx input; Vv input
function R_aero = fcn(ro,Af,Cx,Vv)
R_aero=0.5*(ro*Af*Cx*Vv^2);

== matlab function TrafegabilidadeVerticalAtivo/MOTOR/Torque motor [Nm] ==
  data: Pmax input; T output; wPmax input; w input
function T = fcn(Pmax,wPmax,w)
%Torque JASSAR [Nm]
%________________IMPORTANTE!!!!
%Pmax[W];
%w[rad/s];
if w==0
    T=0;
else
    Pma=1000*Pmax;   %Converção de kW a W.
    wmax=wPmax*pi/30; %Converção de rpm a rad/s.
    P1=0.87*Pma/wmax;
    P2=1.13*Pma/(wmax)^2;
    P3=-Pma/(wmax)^3;
    T=P1+P2*w+P3*w^2;
end
end

== matlab function TrafegabilidadeVerticalAtivo/Rolamento/DISTRIBUIÇÃO DO PESO /Transf Dinâmica Peso ==
  data: a1 input; a2 input; b1 input; b2 input; h_CG input; W1 output; W input; Ws_b input; av input; W2 output; W3 output; Fxi input
% Sistema de Suspensão - Modelos Passivo e Semiativo
% Autor: Jefferson Gomes de Carvalho Souza
function [W1,W2, W3] = fcn(a1,a2,b1,b2, h_CG,W,Ws_b, av, Fxi)
%==============================IMPORTANTE!!!!==============================
%Hipóteses
%1. A dinâmica lateral é do caminhão enteiro (SEIS RODAS)
%2.	O caminhão não têm movimento de mergulho nem de agachamento.
%3.	As alturas dos centros de gravidade do chassis e do bogie são iguais.
%4.	As forças tractivas de cada roda é igual (Ft=6*Fx). 
%==========================================================================
L=a1+a2; %Cumprimento entre eixo dianteiro e cm do bogie.
l=b1+b2; %Cumprimiento entre eixo 2 e eixo 3. 
g=9.81; %Acelaração da gravedade

%Cálculo da reação de ligação no eixo longitudinal x no ponto "T".
Fx_T=W/g*av-2*Fxi;

if av>0||av<0
    if av>0
        
        W1=a2/L*W-(h_CG/L)*(av/g*W-Fx_T); % Reação eixo 1 [N]
        WT=W-W1; %Reação de ligação no eixo z no ponto "T".
        W2=b2/l*(WT+Ws_b)-(h_CG/l)*(av/g*Ws_b+Fx_T);% Reação eixo 2 [N]
        W3=b1/l*(WT+Ws_b)+(h_CG/l)*(av/g*Ws_b+Fx_T);% Reação eixo 3 [N]
     else
    %Equação no caso da aceleração do carro!!! (Signo +,-)
        
        W1=a2/L*W+(h_CG/L)*(av/g*W-Fx_T); % Reação eixo 1 [N]
        WT=W-W1; %Reação de ligação no eixo z no ponto "T".
        W2=b2/l*(WT+Ws_b)+(h_CG/l)*(av/g*Ws_b+Fx_T);% Reação eixo 2 [N]
        W3=b1/l*(WT+Ws_b)-(h_CG/l)*(av/g*Ws_b+Fx_T);% Reação eixo 3 [N]
        
     end
else
    W1=(a2/L)*W; %Reação eixo 1 [N]
    WT=W-W1; %Reação de ligação no eixo z no ponto "T".
    W2=b2/l*(WT+Ws_b); % Reação eixo 2 [N]
    W3=b1/l*(WT+Ws_b); % Reação eixo 3 [N]
end
end

== stateflow chart TrafegabilidadeVerticalAtivo/Motorista/Seletor de marcha ==
  state Primeira_1
    entry: m=1;
  state Segunda_2
    entry: m=2;
  state Terceira_3
    entry: m=3;
  state Quarta_4
    entry: m=4;
  state Quinta_5
    entry: m=5;
  state Sexta_6
    entry: m=6;
  state Decima_12
    entry: m=12;
  state Decima_11
    entry: m=11;
  state Decima_10
    entry: m=10;
  state Nona_9
    entry: m=9;
  state Oitava_8
    entry: m=8;
  state Setima_7
    entry: m=7;
  note: ?
  note: ?
  (default) -> Primeira_1
  Primeira_1 -> Segunda_2 : [v>=6.4]
  Segunda_2 -> Terceira_3 [order 2] : [v>=7.2]
  Terceira_3 -> Quarta_4 [order 2] : [v>=9.3]
  Quarta_4 -> Quinta_5 [order 2] : [v>=11.4]
  Quinta_5 -> Sexta_6 [order 2] : [v>=14.3]
  Setima_7 -> Sexta_6 [order 1] : [v<17.9]
  Sexta_6 -> Setima_7 [order 2] : [v>=17.9]
  Segunda_2 -> Primeira_1 [order 1] : [v<6.4]
  Terceira_3 -> Segunda_2 [order 1] : [v<7.2]
  Quarta_4 -> Terceira_3 [order 1] : [v<9.3]
  Quinta_5 -> Quarta_4 [order 1] : [v<11.4]
  Sexta_6 -> Quinta_5 [order 1] : [v<14.3]
  Decima_11 -> Decima_12 [order 2] : [v>=53]
  Decima_10 -> Decima_11 [order 2] : [v>=42.2]
  Nona_9 -> Decima_10 [order 2] : [v>=34.3]
  Oitava_8 -> Nona_9 [order 2] : [v>=27.2]
  Setima_7 -> Oitava_8 [order 2] : [v>=22.2]
  Decima_12 -> Decima_11 : [v<53]
  Decima_11 -> Decima_10 [order 1] : [v<42.2]
  Decima_10 -> Nona_9 [order 1] : [v<34.3]
  Nona_9 -> Oitava_8 [order 1] : [v<27.2]
  Oitava_8 -> Setima_7 [order 1] : [v<22.2]
  data: v input; m output

== matlab function TrafegabilidadeVerticalAtivo/Suspensão batente eixo 3/SUSPENSÃO BATENTE/Batente da suspensão ==
  data: ks3 input; DeltaZ input; FK3 output
function FK3 = fcn(ks3, DeltaZ)
%% Entradas: DeltaZ(Z3-ZT2) [m] e ZT2 [m] parte traseira.
%% MOLA
%MOLA SUSPENSÃO   [ks] (10000Nm ~ 20000Nm)
%km_rebound=1e+06;   %REBOUND:Constante elástica de mola no caso a roda esteja sem contato.
km_bump=1.5e+06; %BUMP:Constante elástica máxima da mola. 
delta_max=0.7;
if DeltaZ<=delta_max
    FK3=ks3*DeltaZ;
else
    FK3=km_bump*DeltaZ;
end
